simulink model "Control_For_exp3"  (R2015b)
settings: Solver=VariableStepAuto  StartTime=0.0  StopTime=10.0  RelTol=1e-3
StartFcn:
  | open_scope
settings Model: Creator=LUBO  LastModifiedBy=LUBO

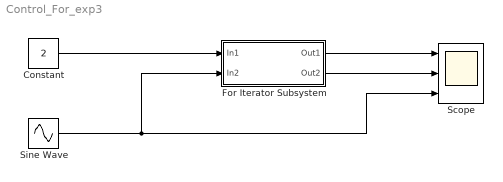
== system Control_For_exp3 ==
  Constant : Constant  Value=2
  For Iterator Subsystem : Subsystem  TreatAsAtomicUnit=on
  Scope : Scope  NumInputPorts=3
  Sine Wave : Sin  Amplitude=11  SampleTime=0
  wires:
  For Iterator Subsystem/1(Out1) -> Scope/1
  Constant/1 -> For Iterator Subsystem/1(In1)
  Sine Wave/1 -> Scope/3, For Iterator Subsystem/2(In2)
  For Iterator Subsystem/2(Out2) -> Scope/2

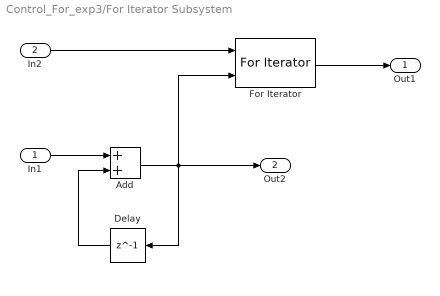
== system Control_For_exp3/For Iterator Subsystem ==
  In1 : Inport
  In2 : Inport  Port=2
  Add : Sum
  Delay : Delay  DelayLength=1  InitialCondition=0
  For Iterator : ForIterator  IterationSource=external  ExternalIncrement=on  IterationVariableDataType=double
  Out1 : Outport
  Out2 : Outport  Port=2
  wires:
  For Iterator/1 -> Out1/1
  In2/1 -> For Iterator/1
  In1/1 -> Add/1
  Add/1 -> For Iterator/2, Delay/1, Out2/1
  Delay/1 -> Add/2
